simulink model "rover_gs"  (R2015a)
settings: Solver=ode4  StartTime=0.0  StopTime=inf  FixedStep=0.01  RelTol=1e-3
libraries: instrumentlib x2, simulink x2
settings Model: Creator=Ssubrama  LastModifiedBy=Aldux
settings DataIOCC: SignalLoggingSaveFormat=ModelDataLogs
settings OptimizationCC: ExpressionDepthLimit=2147483647  InitFltsAndDblsToZero=on
settings DebuggingCC: UnderspecifiedInitializationDetection=Classic  MergeDetectMultiDrivingBlocksExec=none  SolverPrmCheckMsg=warning  MultiTaskDSMMsg=warning  MultiTaskCondExecSysMsg=none  FcnCallInpInsideContextMsg=UseLocalSettings  StateNameClashWarn=warning
settings GRTTargetCC: TargetFcnLib=ansi_tfl_tmw_new.mat  CombineOutputUpdateFcns=off  GRTInterface=on

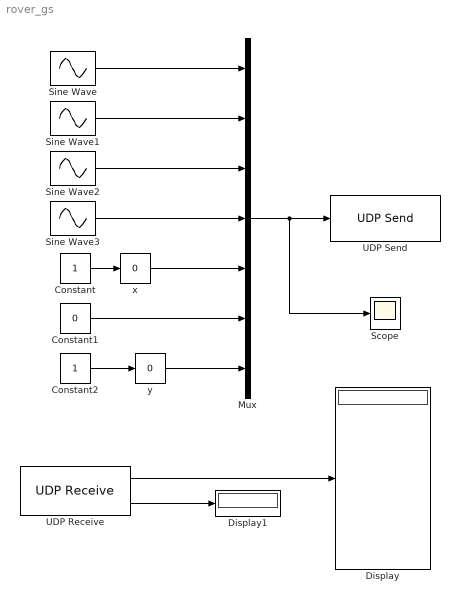
== system rover_gs ==
  Constant : Constant
  Constant1 : Constant  Value=0
  Constant2 : Constant
  Display : Display
  Display1 : Display
  Mux : Mux  Inputs=7
  Scope : Scope
  Sine Wave : Sin  Priority=1  SampleTime=0.01
  Sine Wave1 : Sin  Priority=1  Bias=4  SampleTime=0.01
  Sine Wave2 : Sin  Priority=1  Bias=-2  SampleTime=0.01
  Sine Wave3 : Sin  Priority=1  Amplitude=2  SampleTime=0.01
  UDP Receive : instrumentlib/UDP Receive  Host=localhost  Port=51002  LocalPort=51002  DataSize="[10   1]"  EnableBlockingMode=off  Timeout=10  SampleTime=0.01  DataType=double  ByteOrder=BigEndian
  UDP Send : instrumentlib/UDP Send  Priority=2  Host=localhost  Port=51001  LocalPort=51000  EnableBlockingMode=on  ByteOrder=BigEndian
  x : simulink/Math Operations/Slider Gain  low=-2  gain=0  high=2
  y : simulink/Math Operations/Slider Gain  low=-2  gain=0  high=2
  wires:
  Sine Wave/1 -> Mux/1
  Sine Wave1/1 -> Mux/2
  Sine Wave2/1 -> Mux/3
  Sine Wave3/1 -> Mux/4
  Mux/1 -> Scope/1, UDP Send/1
  Constant/1 -> x/1
  Constant2/1 -> y/1
  x/1 -> Mux/5
  Constant1/1 -> Mux/6
  y/1 -> Mux/7
  UDP Receive/1 -> Display/1
  UDP Receive/2 -> Display1/1
